simulink model "PropulsionTest"  (R2017b)
settings: Solver=FixedStepAuto  StartTime=0.0  StopTime=100*24*60*60  FixedStep=.2  RelTol=1e-3
model workspace: external: MATLAB File C:\Users\Justin\Documents\00 MEng Project\PAN_ADCS\initialization\simulink_workspace_init.m (data not in the file)
undefined symbols (not defined in the file): Imp_max, Imp_min, init, K_F, L_F, m_follower, match_tol, muE, ontime_max, ontime_min, Thrust_max, Thrust_min
libraries: hEemethod x8, vrlib x2, dspsigattribs x1
(part 1 of 2)
settings Model: Creator=Justin  LastModifiedBy=Justin

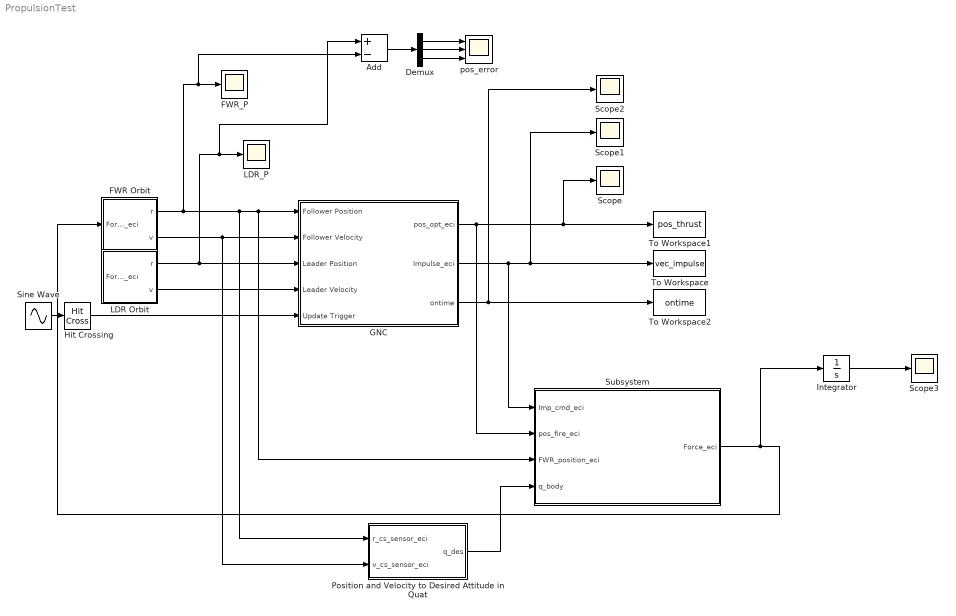
== system PropulsionTest ==
  Add : Sum  Inputs=+-
  Demux : Demux  Outputs=3
  FWR Orbit : Subsystem
  FWR_P : Scope
  GNC : Subsystem
  Hit Crossing : HitCross  HitCrossingOffset=0.5  HitCrossingDirection=rising
  Integrator : Integrator  InitialCondition=[0;0;0]
  LDR Orbit : Subsystem
  LDR_P : Scope
  Position and Velocity to Desired Attitude in Quat : Subsystem
  Scope{,1..3} (4 alike) : Scope
  Sine Wave : Sin  Frequency=2*pi/550  SampleTime=0
  Subsystem : Subsystem
  To Workspace : ToWorkspace  VariableName=vec_impulse  SaveFormat=Timeseries  SampleTime=-1
  To Workspace1 : ToWorkspace  VariableName=pos_thrust  SaveFormat=Timeseries  SampleTime=-1
  To Workspace2 : ToWorkspace  VariableName=ontime  SaveFormat=Timeseries  SampleTime=-1
  pos_error : Scope  NumInputPorts=3
  wires:
  Sine Wave/1 -> Hit Crossing/1
  GNC/3(ontime) -> Scope2/1, To Workspace2/1
  Hit Crossing/1 -> GNC/5(Update Trigger)
  GNC/1(pos_opt_eci) -> Scope/1, To Workspace1/1, Subsystem/2(pos_fire_eci)
  GNC/2(Impulse_eci) -> To Workspace/1, Scope1/1, Subsystem/1(Imp_cmd_eci)
  LDR Orbit/1(r) -> Add/1, LDR_P/1, GNC/3(Leader Position)
  LDR Orbit/2(v) -> GNC/4(Leader Velocity)
  FWR Orbit/2(v) -> Position and Velocity to Desired Attitude in Quat/2(v_cs_sensor_eci), GNC/2(Follower Velocity)
  FWR Orbit/1(r) -> Add/2, FWR_P/1, Position and Velocity to Desired Attitude in Quat/1(r_cs_sensor_eci), Subsystem/3(FWR_position_eci), GNC/1(Follower Position)
  Position and Velocity to Desired Attitude in Quat/1(q_des) -> Subsystem/4(q_body)
  Subsystem/1(Force_eci) -> FWR Orbit/1(Force_eci), Integrator/1
  Integrator/1 -> Scope3/1
  Add/1 -> Demux/1
  Demux/2 -> pos_error/2
  Demux/3 -> pos_error/3
  Demux/1 -> pos_error/1

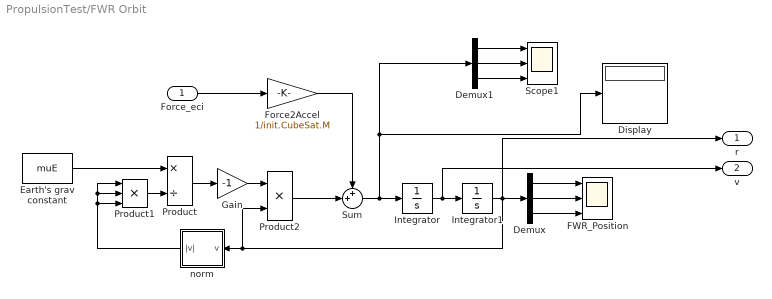
== system PropulsionTest/FWR Orbit ==
  Force_eci : Inport
  Demux : Demux  Outputs=3
  Demux1 : Demux  Outputs=3
  Display : Display
  Earth's grav constant : Constant  Value=muE
  FWR_Position : Scope  NumInputPorts=3
  Force2Accel : Gain  Gain=1/init.CubeSat.M
  Gain : Gain  Gain=-1  SaturateOnIntegerOverflow=on  OutDataTypeStr=Inherit: Same as input  ParamDataTypeStr=Inherit: Same as input
  Integrator : Integrator  InitialCondition=init.FWR.V
  Integrator1 : Integrator  InitialCondition=init.FWR.P
  Product : Product  Inputs=*/  SaturateOnIntegerOverflow=on  OutDataTypeStr=Inherit: Same as first input
  Product1 : Product  Inputs=***  SaturateOnIntegerOverflow=on  OutDataTypeStr=Inherit: Same as first input
  Product2 : Product  Inputs=**  SaturateOnIntegerOverflow=on  OutDataTypeStr=Inherit: Same as first input
  Scope1 : Scope  NumInputPorts=3
  Sum : Sum  Inputs=++|
  norm : Subsystem
  r : Outport
  v : Outport  Port=2
  wires:
  norm/1(|v|) -> Product1/3, Product1/2, Product1/1
  Demux/3 -> FWR_Position/3
  Demux/2 -> FWR_Position/2
  Demux/1 -> FWR_Position/1
  Gain/1 -> Product2/1
  Integrator/1 -> v/1, Integrator1/1
  Product/1 -> Gain/1
  Integrator1/1 -> r/1, Demux/1, norm/1(v), Product2/2
  Product1/1 -> Product/2
  Earth's grav constant/1 -> Product/1
  Force2Accel/1 -> Sum/1
  Product2/1 -> Sum/2
  Sum/1 -> Display/1, Demux1/1, Integrator/1
  Force_eci/1 -> Force2Accel/1
  Demux1/2 -> Scope1/2
  Demux1/3 -> Scope1/3
  Demux1/1 -> Scope1/1

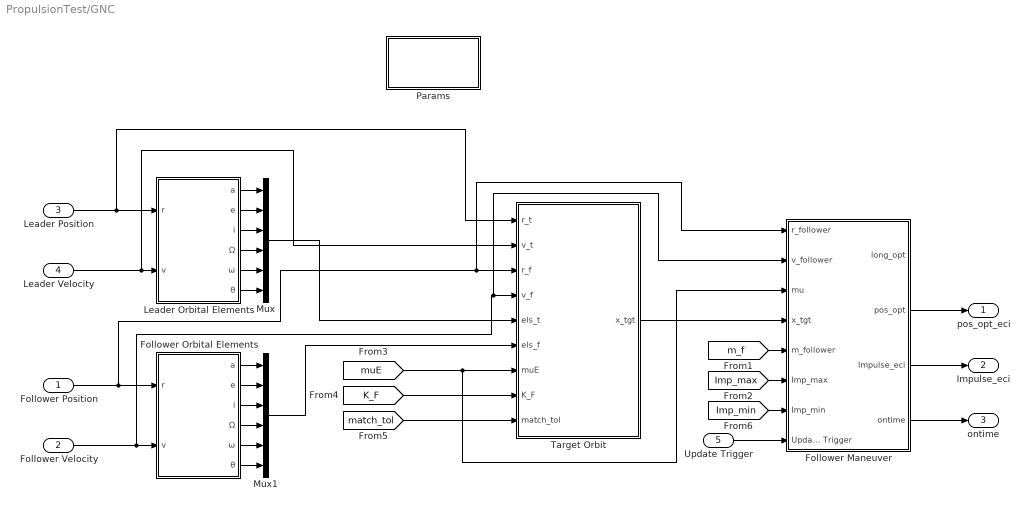
== system PropulsionTest/GNC ==
  Follower Position : Inport
  Follower Velocity : Inport  Port=2
  Leader Position : Inport  Port=3
  Leader Velocity : Inport  Port=4
  Update Trigger : Inport  Port=5
  Follower Maneuver : Subsystem
  Follower Orbital Elements : Subsystem
  Leader Orbital Elements : Subsystem
  Mux : Mux  Inputs=6
  Mux1 : Mux  Inputs=6
  Params : Subsystem
  Target Orbit : MATLAB Function  TreatAsAtomicUnit=on
  pos_opt_eci : Outport
  Impulse_eci : Outport  Port=2
  ontime : Outport  Port=3
  wires:
  Follower Position/1 -> Follower Orbital Elements/1(r), Follower Maneuver/1(r_follower), Target Orbit/3(r_f)
  Follower Maneuver/2(pos_opt) -> pos_opt_eci/1
  [Imp_min] -> Follower Maneuver/7(Imp_min)
  Follower Maneuver/3(Impulse_eci) -> Impulse_eci/1
  Leader Orbital Elements/4(Ω) -> Mux/4
  Mux/1 -> Target Orbit/5(els_t)
  Follower Orbital Elements/6(θ) -> Mux1/6
  Follower Orbital Elements/2(e) -> Mux1/2
  Follower Orbital Elements/3(i) -> Mux1/3
  Update Trigger/1 -> Follower Maneuver/8(Update Trigger)
  Leader Velocity/1 -> Leader Orbital Elements/2(v), Target Orbit/2(v_t)
  [Imp_max] -> Follower Maneuver/6(Imp_max)
  Target Orbit/1(x_tgt) -> Follower Maneuver/4(x_tgt)
  [muE] -> Follower Maneuver/3(mu), Target Orbit/7(muE)
  [match_tol] -> Target Orbit/9(match_tol)
  [m_f] -> Follower Maneuver/5(m_follower)
  Follower Velocity/1 -> Follower Orbital Elements/2(v), Follower Maneuver/2(v_follower), Target Orbit/4(v_f)
  Follower Orbital Elements/1(a) -> Mux1/1
  Follower Orbital Elements/4(Ω) -> Mux1/4
  Leader Orbital Elements/5(ω) -> Mux/5
  Follower Maneuver/4(ontime) -> ontime/1
  Mux1/1 -> Target Orbit/6(els_f)
  Leader Orbital Elements/3(i) -> Mux/3
  Follower Orbital Elements/5(ω) -> Mux1/5
  Leader Orbital Elements/6(θ) -> Mux/6
  Leader Position/1 -> Leader Orbital Elements/1(r), Target Orbit/1(r_t)
  Leader Orbital Elements/1(a) -> Mux/1
  Leader Orbital Elements/2(e) -> Mux/2
  [K_F] -> Target Orbit/8(K_F)

== system PropulsionTest/LDR Orbit ==
  Force_eci : Inport
  Demux : Demux  Outputs=3
  Earth's grav constant : Constant  Value=muE
  Force2Accel : Gain  Gain=1/init.CubeSat.M
  Gain : Gain  Gain=-1  SaturateOnIntegerOverflow=on  OutDataTypeStr=Inherit: Same as input  ParamDataTypeStr=Inherit: Same as input
  Integrator : Integrator  InitialCondition=init.LDR.V
  Integrator1 : Integrator  InitialCondition=init.LDR.P
  LDR_Position : Scope  NumInputPorts=3
  Product : Product  Inputs=*/  SaturateOnIntegerOverflow=on  OutDataTypeStr=Inherit: Same as first input
  Product1 : Product  Inputs=***  SaturateOnIntegerOverflow=on  OutDataTypeStr=Inherit: Same as first input
  Product2 : Product  Inputs=**  SaturateOnIntegerOverflow=on  OutDataTypeStr=Inherit: Same as first input
  Sum : Sum  Inputs=++|
  norm : Subsystem
  r : Outport
  v : Outport  Port=2
  wires:
  norm/1(|v|) -> Product1/3, Product1/2, Product1/1
  Demux/3 -> LDR_Position/3
  Demux/2 -> LDR_Position/2
  Demux/1 -> LDR_Position/1
  Gain/1 -> Product2/1
  Integrator/1 -> v/1, Integrator1/1
  Product/1 -> Gain/1
  Integrator1/1 -> r/1, Demux/1, norm/1(v), Product2/2
  Product1/1 -> Product/2
  Earth's grav constant/1 -> Product/1
  Force2Accel/1 -> Sum/1
  Product2/1 -> Sum/2
  Sum/1 -> Integrator/1
  Force_eci/1 -> Force2Accel/1

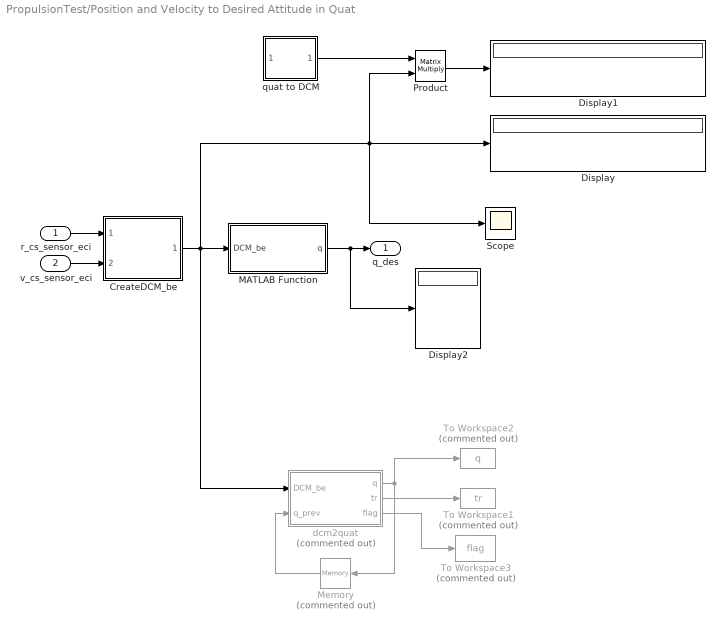
== system PropulsionTest/Position and Velocity to Desired Attitude in Quat ==
  r_cs_sensor_eci : Inport
  v_cs_sensor_eci : Inport  Port=2
  CreateDCM_be : Subsystem
  Display : Display
  Display1 : Display
  Display2 : Display
  MATLAB Function : MATLAB Function  TreatAsAtomicUnit=on
  Memory : Memory  Commented=on
  Product : Product  Multiplication=Matrix(*)
  Scope : Scope
  To Workspace1 : ToWorkspace  Commented=on  VariableName=tr  SampleTime=-1
  To Workspace2 : ToWorkspace  Commented=on  VariableName=q  SampleTime=-1
  To Workspace3 : ToWorkspace  Commented=on  VariableName=flag  SampleTime=-1
  dcm2quat : MATLAB Function  Commented=on  TreatAsAtomicUnit=on
  quat to DCM : Subsystem  mask(Direction Cosine Matrix){}
      mask help: Determines the 3x3 Direction Cosine Matrix (DCM) from a 4x1 quaternion orientation vector. The outputted DCM transforms vectors from inertial axes to body axes. This version corrects the fucked-up MATLAB one.
      mask Help:
      | <p>This block determines the 3x3 Direction Cosine Matrix (DCM) from a 4x1 quaternion orientation vector. The outputted DCM transforms vectors from inertial axes to body axes.  This version corrects the fucked-up MATLAB one</p>
      | 
      | <p>The block input and output contain more than one signal as described below.</p>
      | 
      | <p><H4>Block Vector Input - Quaternion</H4>
      | <ul>
      | <li>q0</li>
      | <li>q1</li>
      | <li>q2</li>
      | <li>q3</li>
      | </ul>
      | </p>
      | 
      | <p><H4>Block Matrix Output - Direction Cosine Matrix  </H4>
      |     <ul>
      |    </ul>
      |    </p>
      mask Display: disp('q to Q')
  q_des : Outport
  wires:
  r_cs_sensor_eci/1 -> CreateDCM_be/1(Position)
  v_cs_sensor_eci/1 -> CreateDCM_be/2(Velocity)
  dcm2quat/1(q) -> Memory/1, To Workspace2/1
  CreateDCM_be/1(DCM_be) -> dcm2quat/1(DCM_be), MATLAB Function/1(DCM_be), Scope/1, Product/2, Display/1
  dcm2quat/2(tr) -> To Workspace1/1
  dcm2quat/3(flag) -> To Workspace3/1
  Memory/1 -> dcm2quat/2(q_prev)
  Product/1 -> Display1/1
  quat to DCM/1(DCM) -> Product/1
  MATLAB Function/1(q) -> Display2/1, q_des/1

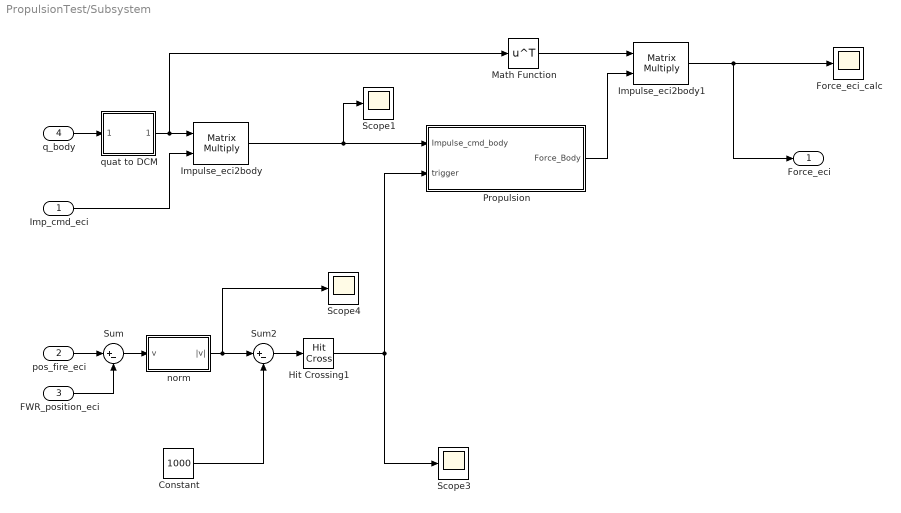
== system PropulsionTest/Subsystem ==
  Imp_cmd_eci : Inport
  pos_fire_eci : Inport  Port=2
  FWR_position_eci : Inport  Port=3
  q_body : Inport  Port=4
  Constant : Constant  Value=1000
  Force_eci_calc : Scope
  Hit Crossing1 : HitCross  HitCrossingDirection=falling
  Impulse_eci2body : Product  Multiplication=Matrix(*)
  Impulse_eci2body1 : Product  Multiplication=Matrix(*)
  Math Function : Math  Operator=transpose  SaturateOnIntegerOverflow=on
  Propulsion : Subsystem
  Scope1 : Scope
  Scope3 : Scope
  Scope4 : Scope
  Sum : Sum  Inputs=|+-
  Sum2 : Sum  Inputs=|+-
  norm : Subsystem
  quat to DCM : Subsystem  mask(Direction Cosine Matrix){}
      mask help: Determines the 3x3 Direction Cosine Matrix (DCM) from a 4x1 quaternion orientation vector. The outputted DCM transforms vectors from inertial axes to body axes. This version corrects the fucked-up MATLAB one.
      mask Help:
      | <p>This block determines the 3x3 Direction Cosine Matrix (DCM) from a 4x1 quaternion orientation vector. The outputted DCM transforms vectors from inertial axes to body axes.  This version corrects the fucked-up MATLAB one</p>
      | 
      | <p>The block input and output contain more than one signal as described below.</p>
      | 
      | <p><H4>Block Vector Input - Quaternion</H4>
      | <ul>
      | <li>q0</li>
      | <li>q1</li>
      | <li>q2</li>
      | <li>q3</li>
      | </ul>
      | </p>
      | 
      | <p><H4>Block Matrix Output - Direction Cosine Matrix  </H4>
      |     <ul>
      |    </ul>
      |    </p>
      mask Display: disp('q to Q')
  Force_eci : Outport
  wires:
  pos_fire_eci/1 -> Sum/1
  FWR_position_eci/1 -> Sum/2
  Sum2/1 -> Hit Crossing1/1
  norm/1(|v|) -> Sum2/1, Scope4/1
  Constant/1 -> Sum2/2
  Sum/1 -> norm/1(v)
  Imp_cmd_eci/1 -> Impulse_eci2body/2
  q_body/1 -> quat to DCM/1(e0 e1 e2 e3)
  Impulse_eci2body/1 -> Scope1/1, Propulsion/1(Impulse_cmd_body)
  Hit Crossing1/1 -> Propulsion/2(trigger), Scope3/1
  Propulsion/1(Force_Body) -> Impulse_eci2body1/2
  quat to DCM/1(DCM) -> Math Function/1, Impulse_eci2body/1
  Math Function/1 -> Impulse_eci2body1/1
  Impulse_eci2body1/1 -> Force_eci/1, Force_eci_calc/1

== system PropulsionTest/FWR Orbit/norm ==
  v : Inport
  Dot Product : DotProduct  InputSameDT=on  OutDataTypeStr=Inherit: Inherit via internal rule
  Math Function : Math  Operator=sqrt  SaturateOnIntegerOverflow=on
  Saturation : Saturate  UpperLimit=1e20  LowerLimit=1e-10
  |v| : Outport
  wires:
  Saturation/1 -> |v|/1
  Math Function/1 -> Saturation/1
  Dot Product/1 -> Math Function/1
  v/1 -> Dot Product/2, Dot Product/1

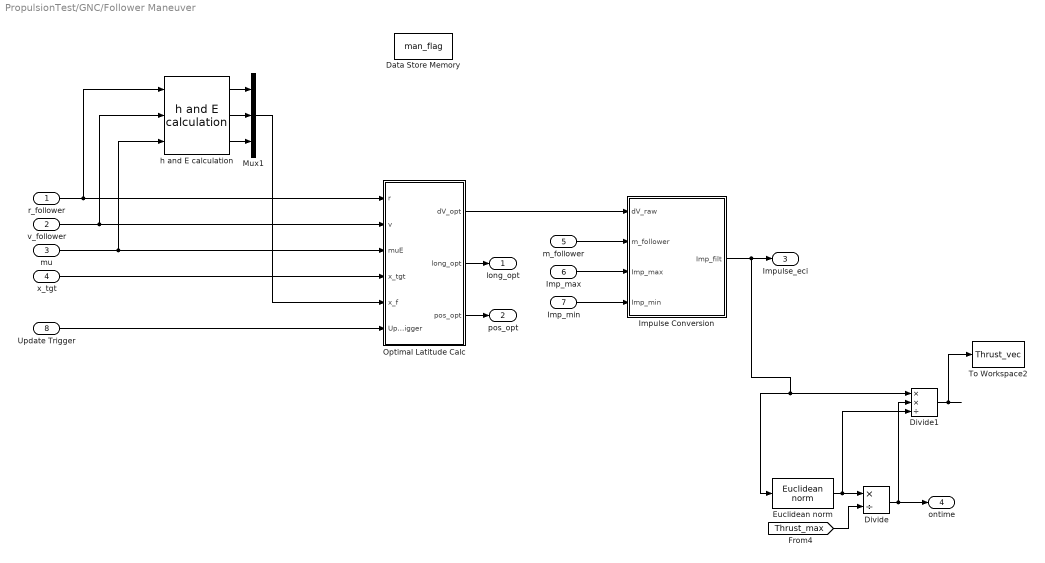
== system PropulsionTest/GNC/Follower Maneuver ==
  r_follower : Inport
  v_follower : Inport  Port=2
  mu : Inport  Port=3
  x_tgt : Inport  Port=4
  m_follower : Inport  Port=5
  Imp_max : Inport  Port=6
  Imp_min : Inport  Port=7
  Update Trigger : Inport  Port=8
  Data Store Memory : DataStoreMemory  DataStoreName=man_flag  WriteAfterWriteMsg=warning  WriteAfterReadMsg=warning  ShowAdditionalParam=off
  Divide : Product  Inputs=*/
  Divide1 : Product  Inputs=**/
  Euclidean norm : hEemethod/Math Operations/Euclidean norm
      settings: SourceProductName=HEe Method Library
  Impulse Conversion : MATLAB Function  TreatAsAtomicUnit=on
  Mux1 : Mux  Inputs=3
  Optimal Latitude Calc : Subsystem
  To Workspace2 : ToWorkspace  VariableName=Thrust_vec  SaveFormat=Timeseries  SampleTime=-1
  h and E calculation : hEemethod/Math Operations/h and E calculation
      settings: SourceProductName=HEe Method Library
  long_opt : Outport
  pos_opt : Outport  Port=2
  Impulse_eci : Outport  Port=3
  ontime : Outport  Port=4
  wires:
  r_follower/1 -> h and E calculation/1, Optimal Latitude Calc/1("r ")
  h and E calculation/1 -> Mux1/1
  h and E calculation/2 -> Mux1/2
  Mux1/1 -> Optimal Latitude Calc/5(x_f)
  x_tgt/1 -> Optimal Latitude Calc/4(x_tgt)
  mu/1 -> h and E calculation/3, Optimal Latitude Calc/3(muE)
  v_follower/1 -> h and E calculation/2, Optimal Latitude Calc/2("v ")
  h and E calculation/3 -> Mux1/3
  Optimal Latitude Calc/2(long_opt) -> long_opt/1
  Optimal Latitude Calc/1(dV_opt) -> Impulse Conversion/1(dV_raw)
  Imp_min/1 -> Impulse Conversion/4(Imp_min)
  Imp_max/1 -> Impulse Conversion/3(Imp_max)
  m_follower/1 -> Impulse Conversion/2(m_follower)
  Update Trigger/1 -> Optimal Latitude Calc/6(Update Trigger)
  Optimal Latitude Calc/3(pos_opt) -> pos_opt/1
  Euclidean norm/1 -> Divide1/3, Divide/1
  Divide1/1 -> To Workspace2/1
  [Thrust_max] -> Divide/2
  Divide/1 -> Divide1/2, ontime/1
  Impulse Conversion/1(Imp_filt) -> Euclidean norm/1, Divide1/1, Impulse_eci/1

== system PropulsionTest/GNC/Follower Orbital Elements ==
  r : Inport
  v : Inport  Port=2
  Follower True Anomaly : hEemethod/Math Operations/True Anomaly
      settings: SourceProductName=HEe Method Library
  Mux : Mux  Inputs=3
  Orbital Elements : hEemethod/Math Operations/Orbital Elements
      settings: SourceProductName=HEe Method Library
  h and E calculation : hEemethod/Math Operations/h and E calculation
      settings: SourceProductName=HEe Method Library
  a : Outport
  e : Outport  Port=2
  i : Outport  Port=3
  Ω : Outport  Port=4
  ω : Outport  Port=5
  θ : Outport  Port=6
  wires:
  h and E calculation/1 -> Mux/1
  Orbital Elements/5 -> ω/1
  Orbital Elements/2 -> e/1
  Orbital Elements/3 -> i/1
  Orbital Elements/1 -> a/1
  r/1 -> Follower True Anomaly/1, h and E calculation/1
  Orbital Elements/4 -> Ω/1
  v/1 -> Follower True Anomaly/2, h and E calculation/2
  Mux/1 -> Orbital Elements/1
  h and E calculation/2 -> Mux/2
  h and E calculation/3 -> Mux/3
  [muE] -> Follower True Anomaly/3, Orbital Elements/2, h and E calculation/3
  Follower True Anomaly/1 -> θ/1

== system PropulsionTest/GNC/Leader Orbital Elements ==
  r : Inport
  v : Inport  Port=2
  Follower True Anomaly : hEemethod/Math Operations/True Anomaly
      settings: SourceProductName=HEe Method Library
  Mux : Mux  Inputs=3
  Orbital Elements : hEemethod/Math Operations/Orbital Elements
      settings: SourceProductName=HEe Method Library
  h and E calculation : hEemethod/Math Operations/h and E calculation
      settings: SourceProductName=HEe Method Library
  a : Outport
  e : Outport  Port=2
  i : Outport  Port=3
  Ω : Outport  Port=4
  ω : Outport  Port=5
  θ : Outport  Port=6
  wires:
  h and E calculation/1 -> Mux/1
  Orbital Elements/5 -> ω/1
  Orbital Elements/2 -> e/1
  Orbital Elements/3 -> i/1
  Orbital Elements/1 -> a/1
  r/1 -> Follower True Anomaly/1, h and E calculation/1
  Orbital Elements/4 -> Ω/1
  v/1 -> Follower True Anomaly/2, h and E calculation/2
  Mux/1 -> Orbital Elements/1
  h and E calculation/2 -> Mux/2
  h and E calculation/3 -> Mux/3
  [muE] -> Follower True Anomaly/3, Orbital Elements/2, h and E calculation/3
  Follower True Anomaly/1 -> θ/1

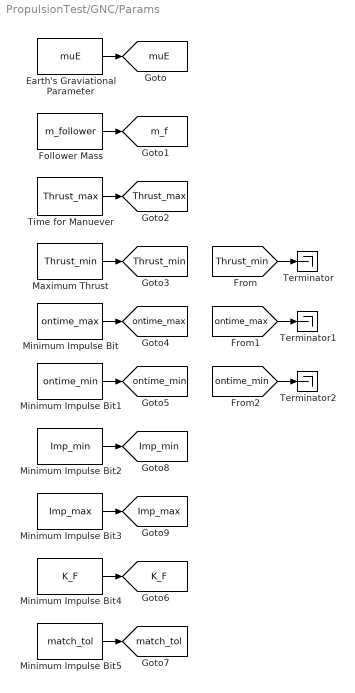
== system PropulsionTest/GNC/Params ==
  Earth's Graviational Parameter : Constant  Value=muE
  Follower Mass : Constant  Value=m_follower
  Maximum Thrust : Constant  Value=Thrust_min
  Minimum Impulse Bit : Constant  Value=ontime_max
  Minimum Impulse Bit1 : Constant  Value=ontime_min
  Minimum Impulse Bit2 : Constant  Value=Imp_min
  Minimum Impulse Bit3 : Constant  Value=Imp_max
  Minimum Impulse Bit4 : Constant  Value=K_F
  Minimum Impulse Bit5 : Constant  Value=match_tol
  Terminator : Terminator
  Terminator1 : Terminator
  Terminator2 : Terminator
  Time for Manuever : Constant  Value=Thrust_max
  tag scope: Imp_max=global, Imp_min=global, K_F=global, Thrust_max=global, Thrust_min=global, m_f=global, match_tol=global, muE=global, ontime_max=global, ontime_min=global
  wires:
  Time for Manuever/1 -> [Thrust_max]
  Follower Mass/1 -> [m_f]
  Earth's Graviational Parameter/1 -> [muE]
  Maximum Thrust/1 -> [Thrust_min]
  Minimum Impulse Bit/1 -> [ontime_max]
  Minimum Impulse Bit1/1 -> [ontime_min]
  Minimum Impulse Bit2/1 -> [Imp_min]
  Minimum Impulse Bit3/1 -> [Imp_max]
  [Thrust_min] -> Terminator/1
  [ontime_max] -> Terminator1/1
  [ontime_min] -> Terminator2/1
  Minimum Impulse Bit4/1 -> [K_F]
  Minimum Impulse Bit5/1 -> [match_tol]

== system PropulsionTest/LDR Orbit/norm ==
  v : Inport
  Dot Product : DotProduct  InputSameDT=on  OutDataTypeStr=Inherit: Inherit via internal rule
  Math Function : Math  Operator=sqrt  SaturateOnIntegerOverflow=on
  Saturation : Saturate  UpperLimit=1e20  LowerLimit=1e-10
  |v| : Outport
  wires:
  Saturation/1 -> |v|/1
  Math Function/1 -> Saturation/1
  Dot Product/1 -> Math Function/1
  v/1 -> Dot Product/2, Dot Product/1

== system PropulsionTest/Position and Velocity to Desired Attitude in Quat/CreateDCM_be ==
  Position : Inport
  Velocity : Inport  Port=2
  Cross Product : vrlib/Utilities/Cross Product
      settings: SourceProductBaseCode=VR
  Cross Product1 : vrlib/Utilities/Cross Product
      settings: SourceProductBaseCode=VR
  Matrix Concatenate : Concatenate  NumInputs=3  Mode=Multidimensional array  ConcatenateDimension=2
  normalize : Subsystem
  normalize2 : Subsystem
  DCM_be : Outport
  wires:
  normalize/1(r_hat) -> Cross Product1/1, Matrix Concatenate/1
  Cross Product/1 -> normalize2/1(v)
  Velocity/1 -> Cross Product/1
  Matrix Concatenate/1 -> DCM_be/1
  Position/1 -> Cross Product/2, normalize/1(r)
  Cross Product1/1 -> Matrix Concatenate/3
  normalize2/1(v_hat) -> Cross Product1/2, Matrix Concatenate/2

== system PropulsionTest/Position and Velocity to Desired Attitude in Quat/quat to DCM ==
  e0 e1 e2 e3 : Inport
  Demux : Demux
  Gain1 : Gain  Gain=2  SaturateOnIntegerOverflow=on  OutDataTypeStr=Inherit: Same as input  ParamDataTypeStr=Inherit: Same as input
  Gain2 : Gain  Gain=2  SaturateOnIntegerOverflow=on  OutDataTypeStr=Inherit: Same as input  ParamDataTypeStr=Inherit: Same as input
  Matrix Gain : Gain  Gain=eye(3,3)  SaturateOnIntegerOverflow=on  OutDataTypeStr=Inherit: Same as input  ParamDataTypeStr=Inherit: Same as input
  Mux : Mux  Inputs=3
  Product : Product  SaturateOnIntegerOverflow=on  InputSameDT=on  OutDataTypeStr=Inherit: Same as first input
  Product1 : Product  SaturateOnIntegerOverflow=on  InputSameDT=on  OutDataTypeStr=Inherit: Same as first input
  Subsystem : Subsystem
      mask Display: disp('3x3 cross matrix')
  Sum1 : Sum  Inputs=|+-  SaturateOnIntegerOverflow=on  InputSameDT=on  OutDataTypeStr=Inherit: Same as first input
  Sum8 : Sum  Inputs=|+-+  SaturateOnIntegerOverflow=on  InputSameDT=on  OutDataTypeStr=Inherit: Same as first input
  T1 : Math  Operator=transpose  SaturateOnIntegerOverflow=on
  T2 : Math  Operator=transpose  SaturateOnIntegerOverflow=on
  qTq : Product  Multiplication=Matrix(*)  SaturateOnIntegerOverflow=on  InputSameDT=on  OutDataTypeStr=Inherit: Same as first input
  qqT : Product  Multiplication=Matrix(*)  SaturateOnIntegerOverflow=on  InputSameDT=on  OutDataTypeStr=Inherit: Same as first input
  DCM : Outport  InitialOutput=0
  wires:
  Subsystem/1(Out1) -> Product/1
  Matrix Gain/1 -> Sum8/3
  Sum1/1 -> Matrix Gain/1
  qTq/1 -> Sum1/2
  T2/1 -> qTq/1
  Product1/1 -> Sum1/1
  Gain1/1 -> Sum8/2
  Gain2/1 -> Sum8/1
  qqT/1 -> Gain2/1
  T1/1 -> qqT/2
  Product/1 -> Gain1/1
  Mux/1 -> qTq/2, T2/1, qqT/1, T1/1, Subsystem/1(In1)
  Demux/4 -> Product1/2, Product1/1, Product/2
  Demux/3 -> Mux/3
  Demux/2 -> Mux/2
  Demux/1 -> Mux/1
  e0 e1 e2 e3/1 -> Demux/1
  Sum8/1 -> DCM/1

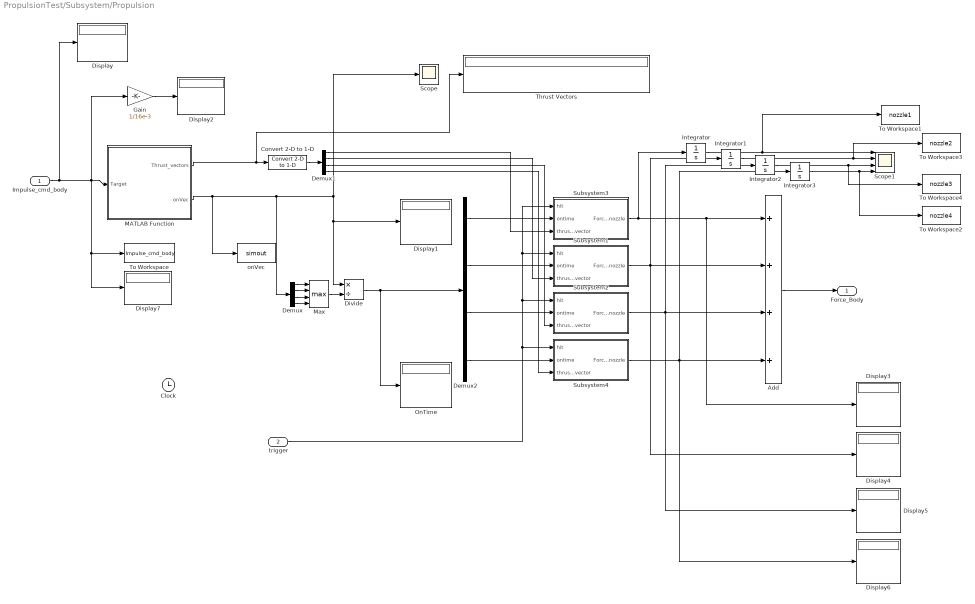
== system PropulsionTest/Subsystem/Propulsion ==
  Impulse_cmd_body : Inport
  trigger : Inport  Port=2
  Add : Sum  Inputs=++++
  Clock : Clock
  Convert 2-D to 1-D : dspsigattribs/Convert 2-D to 1-D
      settings: SourceProductName=DSP System Toolbox  SourceProductBaseCode=DS
  Demux : Demux
  Demux1 : Demux
  Demux2 : Demux
  Display{,1..7} (8 alike) : Display
  Divide : Product  Inputs=*/
  Gain : Gain  Gain=1/16e-3
  Integrator{,1..3} (4 alike) : Integrator  InitialCondition=[0;0;0]
  MATLAB Function : MATLAB Function  TreatAsAtomicUnit=on
  Max : MinMax  Function=max  Inputs=4
  OnTime : Display
  Scope : Scope
  Scope1 : Scope  NumInputPorts=4
  Subsystem1 : Subsystem
  Subsystem2 : Subsystem
  Subsystem3 : Subsystem
  Subsystem4 : Subsystem
  Thrust Vectors : Display
  To Workspace : ToWorkspace  VariableName=Impulse_cmd_body  SaveFormat=Timeseries  SampleTime=-1
  To Workspace1 : ToWorkspace  VariableName=nozzle1  SaveFormat=Timeseries  SampleTime=-1
  To Workspace2 : ToWorkspace  VariableName=nozzle4  SaveFormat=Timeseries  SampleTime=-1
  To Workspace3 : ToWorkspace  VariableName=nozzle2  SaveFormat=Timeseries  SampleTime=-1
  To Workspace4 : ToWorkspace  VariableName=nozzle3  SaveFormat=Timeseries  SampleTime=-1
  onVec : ToWorkspace  VariableName=simout  SaveFormat=Timeseries  SampleTime=-1
  Force_Body : Outport
  wires:
  Impulse_cmd_body/1 -> Display/1, Display7/1, To Workspace/1, Gain/1, MATLAB Function/1(Target)
  MATLAB Function/2(onVec) -> onVec/1, Demux/1, Divide/1, Display1/1, Scope/1
  trigger/1 -> Subsystem4/1(hit), Subsystem2/1(hit), Subsystem1/1(hit), Subsystem3/1(hit)
  Gain/1 -> Display2/1
  Max/1 -> Divide/2
  Divide/1 -> OnTime/1, Demux2/1
  Demux/1 -> Max/1
  Demux/2 -> Max/2
  Demux/3 -> Max/3
  Demux/4 -> Max/4
  Convert 2-D to 1-D/1 -> Demux1/1
  MATLAB Function/1(Thrust_vectors) -> Thrust Vectors/1, Convert 2-D to 1-D/1
  Demux2/1 -> Subsystem3/2(ontime)
  Demux2/2 -> Subsystem1/2(ontime)
  Demux2/3 -> Subsystem2/2(ontime)
  Demux2/4 -> Subsystem4/2(ontime)
  Demux1/1 -> Subsystem3/3(thrust_vector)
  Demux1/2 -> Subsystem1/3(thrust_vector)
  Demux1/3 -> Subsystem2/3(thrust_vector)
  Demux1/4 -> Subsystem4/3(thrust_vector)
  Subsystem3/1(Force_nozzle) -> Integrator/1, Display3/1, Add/1
  Subsystem4/1(Force_nozzle) -> Display6/1, Add/4, Integrator3/1
  Subsystem2/1(Force_nozzle) -> Display5/1, Add/3, Integrator2/1
  Subsystem1/1(Force_nozzle) -> Display4/1, Add/2, Integrator1/1
  Add/1 -> Force_Body/1
  Integrator/1 -> To Workspace1/1, Scope1/1
  Integrator1/1 -> To Workspace3/1, Scope1/2
  Integrator2/1 -> To Workspace4/1, Scope1/3
  Integrator3/1 -> To Workspace2/1, Scope1/4

== system PropulsionTest/Subsystem/norm ==
  v : Inport
  Dot Product : DotProduct  InputSameDT=on  OutDataTypeStr=Inherit: Inherit via internal rule
  Math Function : Math  Operator=sqrt  SaturateOnIntegerOverflow=on
  |v| : Outport
  wires:
  Math Function/1 -> |v|/1
  Dot Product/1 -> Math Function/1
  v/1 -> Dot Product/2, Dot Product/1

== system PropulsionTest/Subsystem/quat to DCM ==
  e0 e1 e2 e3 : Inport
  Demux : Demux
  Gain1 : Gain  Gain=2  SaturateOnIntegerOverflow=on  OutDataTypeStr=Inherit: Same as input  ParamDataTypeStr=Inherit: Same as input
  Gain2 : Gain  Gain=2  SaturateOnIntegerOverflow=on  OutDataTypeStr=Inherit: Same as input  ParamDataTypeStr=Inherit: Same as input
  Matrix Gain : Gain  Gain=eye(3,3)  SaturateOnIntegerOverflow=on  OutDataTypeStr=Inherit: Same as input  ParamDataTypeStr=Inherit: Same as input
  Mux : Mux  Inputs=3
  Product : Product  SaturateOnIntegerOverflow=on  InputSameDT=on  OutDataTypeStr=Inherit: Same as first input
  Product1 : Product  SaturateOnIntegerOverflow=on  InputSameDT=on  OutDataTypeStr=Inherit: Same as first input
  Subsystem : Subsystem
      mask Display: disp('3x3 cross matrix')
  Sum1 : Sum  Inputs=|+-  SaturateOnIntegerOverflow=on  InputSameDT=on  OutDataTypeStr=Inherit: Same as first input
  Sum8 : Sum  Inputs=|+-+  SaturateOnIntegerOverflow=on  InputSameDT=on  OutDataTypeStr=Inherit: Same as first input
  T1 : Math  Operator=transpose  SaturateOnIntegerOverflow=on
  T2 : Math  Operator=transpose  SaturateOnIntegerOverflow=on
  qTq : Product  Multiplication=Matrix(*)  SaturateOnIntegerOverflow=on  InputSameDT=on  OutDataTypeStr=Inherit: Same as first input
  qqT : Product  Multiplication=Matrix(*)  SaturateOnIntegerOverflow=on  InputSameDT=on  OutDataTypeStr=Inherit: Same as first input
  DCM : Outport  InitialOutput=0
  wires:
  Sum8/1 -> DCM/1
  e0 e1 e2 e3/1 -> Demux/1
  Demux/1 -> Mux/1
  Demux/2 -> Mux/2
  Demux/3 -> Mux/3
  Demux/4 -> Product/2, Product1/1, Product1/2
  Mux/1 -> T1/1, qqT/1, Subsystem/1(In1), T2/1, qTq/2
  Product/1 -> Gain1/1
  T1/1 -> qqT/2
  qqT/1 -> Gain2/1
  Gain2/1 -> Sum8/1
  Gain1/1 -> Sum8/2
  Product1/1 -> Sum1/1
  T2/1 -> qTq/1
  qTq/1 -> Sum1/2
  Sum1/1 -> Matrix Gain/1
  Matrix Gain/1 -> Sum8/3
  Subsystem/1(Out1) -> Product/1

== system PropulsionTest/GNC/Follower Maneuver/Optimal Latitude Calc ==
  "r " : Inport
  "v " : Inport  Port=2
  muE : Inport  Port=3
  x_tgt : Inport  Port=4
  x_f : Inport  Port=5
  Update Trigger : Inport  Port=6
  Constant : Constant  Value=K_F
  Constant1 : Constant  Value=L_F
  Enabled Subsystem : Subsystem  TreatAsAtomicUnit=on
  dV_opt : Outport
  long_opt : Outport  Port=2
  pos_opt : Outport  Port=3
  wires:
  Enabled Subsystem/2(long_opt) -> long_opt/1
  "r "/1 -> Enabled Subsystem/1(r)
  "v "/1 -> Enabled Subsystem/2(v)
  muE/1 -> Enabled Subsystem/7("muE ")
  x_tgt/1 -> Enabled Subsystem/3(x_tgt)
  x_f/1 -> Enabled Subsystem/4(x_f)
  Constant/1 -> Enabled Subsystem/5(K)
  Constant1/1 -> Enabled Subsystem/6(L)
  Enabled Subsystem/1(dV_opt) -> dV_opt/1
  Enabled Subsystem/3(pos_opt) -> pos_opt/1
  Update Trigger/1 -> Enabled Subsystem/Enable

== system PropulsionTest/Position and Velocity to Desired Attitude in Quat/CreateDCM_be/normalize ==
  r : Inport
  Dot Product : DotProduct  InputSameDT=on  OutDataTypeStr=Inherit: Inherit via internal rule
  Math Function : Math  Operator=sqrt  SaturateOnIntegerOverflow=on
  Product : Product  Inputs=*/  SaturateOnIntegerOverflow=on  InputSameDT=on  OutDataTypeStr=Inherit: Same as first input
  r_hat : Outport
  wires:
  r/1 -> Dot Product/1, Dot Product/2, Product/1
  Dot Product/1 -> Math Function/1
  Math Function/1 -> Product/2
  Product/1 -> r_hat/1

== system PropulsionTest/Position and Velocity to Desired Attitude in Quat/CreateDCM_be/normalize2 ==
  v : Inport
  Dot Product : DotProduct  InputSameDT=on  OutDataTypeStr=Inherit: Inherit via internal rule
  Math Function : Math  Operator=sqrt  SaturateOnIntegerOverflow=on
  Product : Product  Inputs=*/  SaturateOnIntegerOverflow=on  InputSameDT=on  OutDataTypeStr=Inherit: Same as first input
  v_hat : Outport
  wires:
  v/1 -> Dot Product/1, Dot Product/2, Product/1
  Dot Product/1 -> Math Function/1
  Math Function/1 -> Product/2
  Product/1 -> v_hat/1

== system PropulsionTest/Position and Velocity to Desired Attitude in Quat/quat to DCM/Subsystem ==
  In1 : Inport
  3x3 : Reshape  OutputDimensionality=Customize  OutputDimensions=[3,3]
  Demux : Demux  Outputs=3
  Gain : Gain  Gain=-1  SaturateOnIntegerOverflow=on  OutDataTypeStr=Inherit: Same as input  ParamDataTypeStr=Inherit: Same as input
  Gain1 : Gain  Gain=-1  SaturateOnIntegerOverflow=on  OutDataTypeStr=Inherit: Same as input  ParamDataTypeStr=Inherit: Same as input
  Gain2 : Gain  Gain=-1  SaturateOnIntegerOverflow=on  OutDataTypeStr=Inherit: Same as input  ParamDataTypeStr=Inherit: Same as input
  Mux : Mux  Inputs=9
  "diag 0 " : Constant  Value=0
  Out1 : Outport
  wires:
  Gain2/1 -> Mux/8
  Demux/1 -> Gain2/1, Mux/6
  Gain1/1 -> Mux/4
  Demux/2 -> Mux/7, Gain/1
  Gain/1 -> Mux/3
  Demux/3 -> Gain1/1, Mux/2
  Mux/1 -> 3x3/1
  "diag 0 "/1 -> Mux/9, Mux/5, Mux/1
  3x3/1 -> Out1/1
  In1/1 -> Demux/1

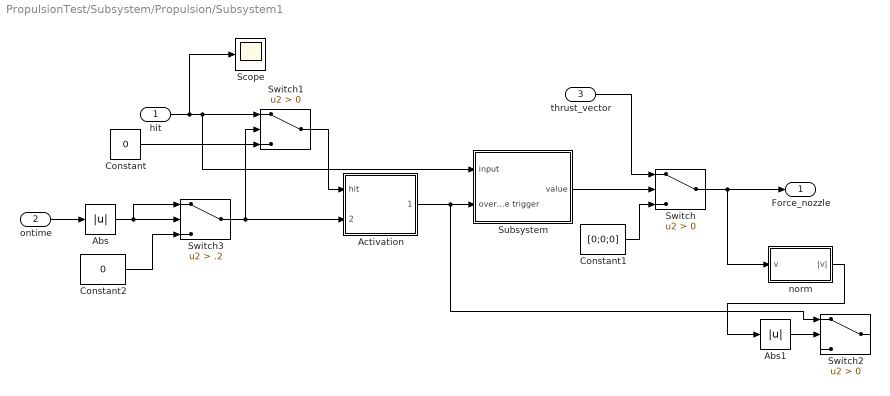
== system PropulsionTest/Subsystem/Propulsion/Subsystem1 ==
  hit : Inport
  ontime : Inport  Port=2
  thrust_vector : Inport  Port=3
  Abs : Abs
  Abs1 : Abs
  Activation : Subsystem
  Constant : Constant  Value=0
  Constant1 : Constant  Value=[0;0;0]
  Constant2 : Constant  Value=0
  Scope : Scope
  Subsystem : Subsystem
  Switch : Switch  Criteria=u2 > Threshold
  Switch1 : Switch  Criteria=u2 > Threshold
  Switch2 : Switch  Criteria=u2 > Threshold
  Switch3 : Switch  Criteria=u2 > Threshold  Threshold=.2
  norm : Subsystem
  Force_nozzle : Outport
  wires:
  Switch3/1 -> Switch1/2, Activation/2(T_maneuver)
  Constant2/1 -> Switch3/3
  ontime/1 -> Abs/1
  hit/1 -> Scope/1, Subsystem/1(input), Switch1/1
  Switch/1 -> norm/1(v), Force_nozzle/1
  Activation/1(man_end) -> Switch2/1, Subsystem/2(overwrite trigger)
  thrust_vector/1 -> Switch/1
  Subsystem/1(value) -> Switch/2
  Constant1/1 -> Switch/3
  Abs/1 -> Switch3/2, Switch3/1
  Switch1/1 -> Activation/1(hit)
  Constant/1 -> Switch1/3
  Abs1/1 -> Switch2/2
  norm/1(|v|) -> Abs1/1

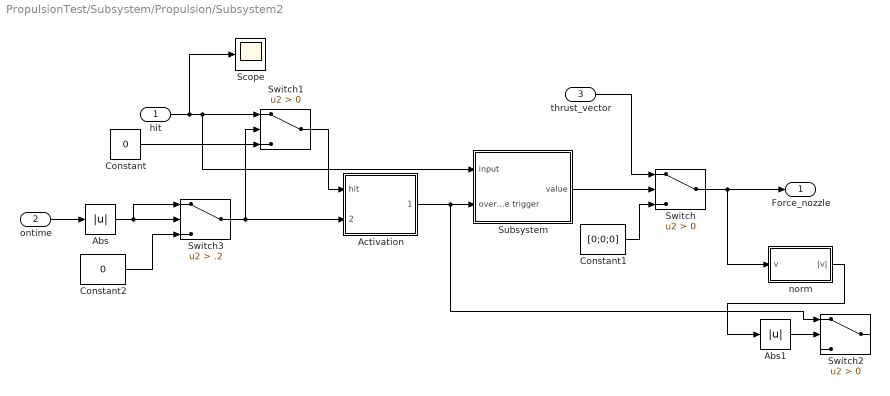
== system PropulsionTest/Subsystem/Propulsion/Subsystem2 ==
  hit : Inport
  ontime : Inport  Port=2
  thrust_vector : Inport  Port=3
  Abs : Abs
  Abs1 : Abs
  Activation : Subsystem
  Constant : Constant  Value=0
  Constant1 : Constant  Value=[0;0;0]
  Constant2 : Constant  Value=0
  Scope : Scope
  Subsystem : Subsystem
  Switch : Switch  Criteria=u2 > Threshold
  Switch1 : Switch  Criteria=u2 > Threshold
  Switch2 : Switch  Criteria=u2 > Threshold
  Switch3 : Switch  Criteria=u2 > Threshold  Threshold=.2
  norm : Subsystem
  Force_nozzle : Outport
  wires:
  norm/1(|v|) -> Abs1/1
  Abs1/1 -> Switch2/2
  Constant/1 -> Switch1/3
  Switch1/1 -> Activation/1(hit)
  Abs/1 -> Switch3/1, Switch3/2
  Constant1/1 -> Switch/3
  Subsystem/1(value) -> Switch/2
  thrust_vector/1 -> Switch/1
  Activation/1(man_end) -> Subsystem/2(overwrite trigger), Switch2/1
  Switch/1 -> Force_nozzle/1, norm/1(v)
  hit/1 -> Switch1/1, Subsystem/1(input), Scope/1
  ontime/1 -> Abs/1
  Constant2/1 -> Switch3/3
  Switch3/1 -> Activation/2(T_maneuver), Switch1/2

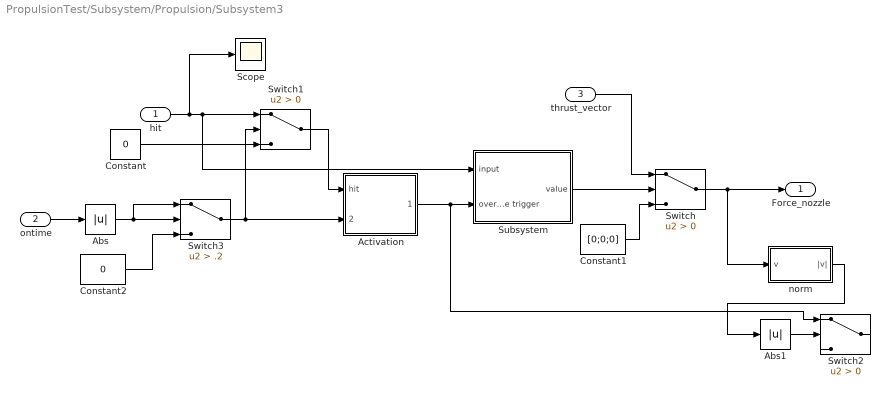
== system PropulsionTest/Subsystem/Propulsion/Subsystem3 ==
  hit : Inport
  ontime : Inport  Port=2
  thrust_vector : Inport  Port=3
  Abs : Abs
  Abs1 : Abs
  Activation : Subsystem
  Constant : Constant  Value=0
  Constant1 : Constant  Value=[0;0;0]
  Constant2 : Constant  Value=0
  Scope : Scope
  Subsystem : Subsystem
  Switch : Switch  Criteria=u2 > Threshold
  Switch1 : Switch  Criteria=u2 > Threshold
  Switch2 : Switch  Criteria=u2 > Threshold
  Switch3 : Switch  Criteria=u2 > Threshold  Threshold=.2
  norm : Subsystem
  Force_nozzle : Outport
  wires:
  norm/1(|v|) -> Abs1/1
  Abs1/1 -> Switch2/2
  Constant/1 -> Switch1/3
  Switch1/1 -> Activation/1(hit)
  Abs/1 -> Switch3/1, Switch3/2
  Constant1/1 -> Switch/3
  Subsystem/1(value) -> Switch/2
  thrust_vector/1 -> Switch/1
  Activation/1(man_end) -> Subsystem/2(overwrite trigger), Switch2/1
  Switch/1 -> Force_nozzle/1, norm/1(v)
  hit/1 -> Switch1/1, Subsystem/1(input), Scope/1
  ontime/1 -> Abs/1
  Constant2/1 -> Switch3/3
  Switch3/1 -> Activation/2(T_maneuver), Switch1/2

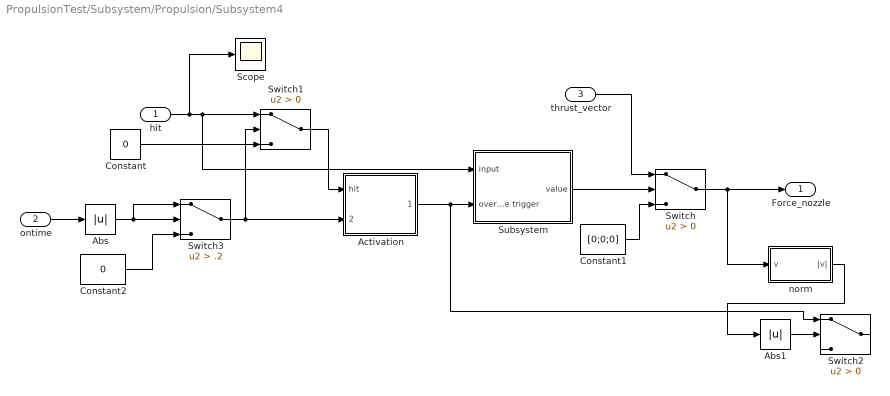
== system PropulsionTest/Subsystem/Propulsion/Subsystem4 ==
  hit : Inport
  ontime : Inport  Port=2
  thrust_vector : Inport  Port=3
  Abs : Abs
  Abs1 : Abs
  Activation : Subsystem
  Constant : Constant  Value=0
  Constant1 : Constant  Value=[0;0;0]
  Constant2 : Constant  Value=0
  Scope : Scope
  Subsystem : Subsystem
  Switch : Switch  Criteria=u2 > Threshold
  Switch1 : Switch  Criteria=u2 > Threshold
  Switch2 : Switch  Criteria=u2 > Threshold
  Switch3 : Switch  Criteria=u2 > Threshold  Threshold=.2
  norm : Subsystem
  Force_nozzle : Outport
  wires:
  Switch3/1 -> Switch1/2, Activation/2(T_maneuver)
  Constant2/1 -> Switch3/3
  ontime/1 -> Abs/1
  hit/1 -> Scope/1, Subsystem/1(input), Switch1/1
  Switch/1 -> norm/1(v), Force_nozzle/1
  Activation/1(man_end) -> Switch2/1, Subsystem/2(overwrite trigger)
  thrust_vector/1 -> Switch/1
  Subsystem/1(value) -> Switch/2
  Constant1/1 -> Switch/3
  Abs/1 -> Switch3/2, Switch3/1
  Switch1/1 -> Activation/1(hit)
  Constant/1 -> Switch1/3
  Abs1/1 -> Switch2/2
  norm/1(|v|) -> Abs1/1

== system PropulsionTest/Subsystem/quat to DCM/Subsystem ==
  In1 : Inport
  3x3 : Reshape  OutputDimensionality=Customize  OutputDimensions=[3,3]
  Demux : Demux  Outputs=3
  Gain : Gain  Gain=-1  SaturateOnIntegerOverflow=on  OutDataTypeStr=Inherit: Same as input  ParamDataTypeStr=Inherit: Same as input
  Gain1 : Gain  Gain=-1  SaturateOnIntegerOverflow=on  OutDataTypeStr=Inherit: Same as input  ParamDataTypeStr=Inherit: Same as input
  Gain2 : Gain  Gain=-1  SaturateOnIntegerOverflow=on  OutDataTypeStr=Inherit: Same as input  ParamDataTypeStr=Inherit: Same as input
  Mux : Mux  Inputs=9
  "diag 0 " : Constant  Value=0
  Out1 : Outport
  wires:
  In1/1 -> Demux/1
  3x3/1 -> Out1/1
  "diag 0 "/1 -> Mux/1, Mux/5, Mux/9
  Mux/1 -> 3x3/1
  Demux/3 -> Mux/2, Gain1/1
  Gain/1 -> Mux/3
  Demux/2 -> Gain/1, Mux/7
  Gain1/1 -> Mux/4
  Demux/1 -> Mux/6, Gain2/1
  Gain2/1 -> Mux/8

== system PropulsionTest/GNC/Follower Maneuver/Optimal Latitude Calc/Enabled Subsystem ==
  r : Inport
  v : Inport  Port=2
  x_tgt : Inport  Port=3
  x_f : Inport  Port=4
  K : Inport  Port=5
  L : Inport  Port=6
  "muE " : Inport  Port=7
  Enable : EnablePort
  MATLAB Function : MATLAB Function  TreatAsAtomicUnit=on
  dV_opt : Outport
  long_opt : Outport  Port=2
  pos_opt : Outport  Port=3
  wires:
  r/1 -> MATLAB Function/1(r)
  v/1 -> MATLAB Function/2(v)
  "muE "/1 -> MATLAB Function/7(muE)
  x_tgt/1 -> MATLAB Function/3(x_t)
  x_f/1 -> MATLAB Function/4(x)
  K/1 -> MATLAB Function/5(K)
  L/1 -> MATLAB Function/6(L)
  MATLAB Function/3(long_opt) -> long_opt/1
  MATLAB Function/1(dV_opt) -> dV_opt/1
  MATLAB Function/2(pos_opt) -> pos_opt/1

== system PropulsionTest/Subsystem/Propulsion/Subsystem1/Activation ==
  note: t_trig + onTime
  note: time of trigger
  note: current time
  hit : Inport
  T_maneuver : Inport  Port=2
  Add : Sum
  Clock : Clock
  Hit Crossing : HitCross
  Subsystem : Subsystem
  Subsystem1 : Subsystem
  Subtract : Sum  Inputs=+-
  man_end : Outport
  wires:
  Subtract/1 -> Hit Crossing/1
  Add/1 -> Subtract/2
  Subsystem/1(value) -> Add/1
  T_maneuver/1 -> Subsystem1/1(input)
  Hit Crossing/1 -> man_end/1
  hit/1 -> Subsystem1/2(overwrite trigger), Subsystem/2(overwrite trigger)
  Clock/1 -> Subtract/1, Subsystem/1(input)
  Subsystem1/1(value) -> Add/2

== system PropulsionTest/Subsystem/Propulsion/Subsystem1/Subsystem ==
  input : Inport
  overwrite trigger : Inport  Port=2
  Data Store Memory : DataStoreMemory  DataStoreName=Mem  ShowAdditionalParam=off
  Data Store Read : DataStoreRead  DataStoreName=Mem  SampleTime=[0,0]  DataStoreElements=Mem
  Data Store Write : DataStoreWrite  DataStoreName=Mem  SampleTime=[0,0]  DataStoreElements=Mem
  Switch : Switch  Criteria=u2 > Threshold
  value : Outport
  wires:
  overwrite trigger/1 -> Switch/2
  Data Store Read/1 -> Switch/3
  Switch/1 -> value/1, Data Store Write/1
  input/1 -> Switch/1

== system PropulsionTest/Subsystem/Propulsion/Subsystem1/norm ==
  v : Inport
  Dot Product : DotProduct  InputSameDT=on  OutDataTypeStr=Inherit: Inherit via internal rule
  Math Function : Math  Operator=sqrt  SaturateOnIntegerOverflow=on
  |v| : Outport
  wires:
  Math Function/1 -> |v|/1
  Dot Product/1 -> Math Function/1
  v/1 -> Dot Product/2, Dot Product/1

== system PropulsionTest/Subsystem/Propulsion/Subsystem2/Activation ==
  note: current time
  note: time of trigger
  note: t_trig + onTime
  hit : Inport
  T_maneuver : Inport  Port=2
  Add : Sum
  Clock : Clock
  Hit Crossing : HitCross
  Subsystem : Subsystem
  Subsystem1 : Subsystem
  Subtract : Sum  Inputs=+-
  man_end : Outport
  wires:
  Subsystem1/1(value) -> Add/2
  Clock/1 -> Subsystem/1(input), Subtract/1
  hit/1 -> Subsystem/2(overwrite trigger), Subsystem1/2(overwrite trigger)
  Hit Crossing/1 -> man_end/1
  T_maneuver/1 -> Subsystem1/1(input)
  Subsystem/1(value) -> Add/1
  Add/1 -> Subtract/2
  Subtract/1 -> Hit Crossing/1

== system PropulsionTest/Subsystem/Propulsion/Subsystem2/Subsystem ==
  input : Inport
  overwrite trigger : Inport  Port=2
  Data Store Memory : DataStoreMemory  DataStoreName=Mem  ShowAdditionalParam=off
  Data Store Read : DataStoreRead  DataStoreName=Mem  SampleTime=[0,0]  DataStoreElements=Mem
  Data Store Write : DataStoreWrite  DataStoreName=Mem  SampleTime=[0,0]  DataStoreElements=Mem
  Switch : Switch  Criteria=u2 > Threshold
  value : Outport
  wires:
  input/1 -> Switch/1
  Switch/1 -> Data Store Write/1, value/1
  Data Store Read/1 -> Switch/3
  overwrite trigger/1 -> Switch/2

== system PropulsionTest/Subsystem/Propulsion/Subsystem2/norm ==
  v : Inport
  Dot Product : DotProduct  InputSameDT=on  OutDataTypeStr=Inherit: Inherit via internal rule
  Math Function : Math  Operator=sqrt  SaturateOnIntegerOverflow=on
  |v| : Outport
  wires:
  v/1 -> Dot Product/1, Dot Product/2
  Dot Product/1 -> Math Function/1
  Math Function/1 -> |v|/1

== system PropulsionTest/Subsystem/Propulsion/Subsystem3/Activation ==
  note: current time
  note: time of trigger
  note: t_trig + onTime
  hit : Inport
  T_maneuver : Inport  Port=2
  Add : Sum
  Clock : Clock
  Hit Crossing : HitCross
  Subsystem : Subsystem
  Subsystem1 : Subsystem
  Subtract : Sum  Inputs=+-
  man_end : Outport
  wires:
  Subsystem1/1(value) -> Add/2
  Clock/1 -> Subsystem/1(input), Subtract/1
  hit/1 -> Subsystem/2(overwrite trigger), Subsystem1/2(overwrite trigger)
  Hit Crossing/1 -> man_end/1
  T_maneuver/1 -> Subsystem1/1(input)
  Subsystem/1(value) -> Add/1
  Add/1 -> Subtract/2
  Subtract/1 -> Hit Crossing/1

== system PropulsionTest/Subsystem/Propulsion/Subsystem3/Subsystem ==
  input : Inport
  overwrite trigger : Inport  Port=2
  Data Store Memory : DataStoreMemory  DataStoreName=Mem  ShowAdditionalParam=off
  Data Store Read : DataStoreRead  DataStoreName=Mem  SampleTime=[0,0]  DataStoreElements=Mem
  Data Store Write : DataStoreWrite  DataStoreName=Mem  SampleTime=[0,0]  DataStoreElements=Mem
  Switch : Switch  Criteria=u2 > Threshold
  value : Outport
  wires:
  input/1 -> Switch/1
  Switch/1 -> Data Store Write/1, value/1
  Data Store Read/1 -> Switch/3
  overwrite trigger/1 -> Switch/2

== system PropulsionTest/Subsystem/Propulsion/Subsystem3/norm ==
  v : Inport
  Dot Product : DotProduct  InputSameDT=on  OutDataTypeStr=Inherit: Inherit via internal rule
  Math Function : Math  Operator=sqrt  SaturateOnIntegerOverflow=on
  |v| : Outport
  wires:
  v/1 -> Dot Product/1, Dot Product/2
  Dot Product/1 -> Math Function/1
  Math Function/1 -> |v|/1

== system PropulsionTest/Subsystem/Propulsion/Subsystem4/Activation ==
  note: t_trig + onTime
  note: time of trigger
  note: current time
  hit : Inport
  T_maneuver : Inport  Port=2
  Add : Sum
  Clock : Clock
  Hit Crossing : HitCross
  Subsystem : Subsystem
  Subsystem1 : Subsystem
  Subtract : Sum  Inputs=+-
  man_end : Outport
  wires:
  Subtract/1 -> Hit Crossing/1
  Add/1 -> Subtract/2
  Subsystem/1(value) -> Add/1
  T_maneuver/1 -> Subsystem1/1(input)
  Hit Crossing/1 -> man_end/1
  hit/1 -> Subsystem1/2(overwrite trigger), Subsystem/2(overwrite trigger)
  Clock/1 -> Subtract/1, Subsystem/1(input)
  Subsystem1/1(value) -> Add/2

== system PropulsionTest/Subsystem/Propulsion/Subsystem4/Subsystem ==
  input : Inport
  overwrite trigger : Inport  Port=2
  Data Store Memory : DataStoreMemory  DataStoreName=Mem  ShowAdditionalParam=off
  Data Store Read : DataStoreRead  DataStoreName=Mem  SampleTime=[0,0]  DataStoreElements=Mem
  Data Store Write : DataStoreWrite  DataStoreName=Mem  SampleTime=[0,0]  DataStoreElements=Mem
  Switch : Switch  Criteria=u2 > Threshold
  value : Outport
  wires:
  overwrite trigger/1 -> Switch/2
  Data Store Read/1 -> Switch/3
  Switch/1 -> value/1, Data Store Write/1
  input/1 -> Switch/1

== system PropulsionTest/Subsystem/Propulsion/Subsystem4/norm ==
  v : Inport
  Dot Product : DotProduct  InputSameDT=on  OutDataTypeStr=Inherit: Inherit via internal rule
  Math Function : Math  Operator=sqrt  SaturateOnIntegerOverflow=on
  |v| : Outport
  wires:
  Math Function/1 -> |v|/1
  Dot Product/1 -> Math Function/1
  v/1 -> Dot Product/2, Dot Product/1

== system PropulsionTest/Subsystem/Propulsion/Subsystem1/Activation/Subsystem ==
  input : Inport
  overwrite trigger : Inport  Port=2
  Data Store Memory : DataStoreMemory  DataStoreName=Mem  ShowAdditionalParam=off
  Data Store Read : DataStoreRead  DataStoreName=Mem  SampleTime=[0,0]  DataStoreElements=Mem
  Data Store Write : DataStoreWrite  DataStoreName=Mem  SampleTime=[0,0]  DataStoreElements=Mem
  Switch : Switch  Criteria=u2 > Threshold
  value : Outport
  wires:
  overwrite trigger/1 -> Switch/2
  Data Store Read/1 -> Switch/3
  Switch/1 -> Data Store Write/1, value/1
  input/1 -> Switch/1

== system PropulsionTest/Subsystem/Propulsion/Subsystem1/Activation/Subsystem1 ==
  input : Inport
  overwrite trigger : Inport  Port=2
  Data Store Memory : DataStoreMemory  DataStoreName=Mem  ShowAdditionalParam=off
  Data Store Read : DataStoreRead  DataStoreName=Mem  SampleTime=[0,0]  DataStoreElements=Mem
  Data Store Write : DataStoreWrite  DataStoreName=Mem  SampleTime=[0,0]  DataStoreElements=Mem
  Switch : Switch  Criteria=u2 > Threshold
  value : Outport
  wires:
  input/1 -> Switch/1
  Switch/1 -> value/1, Data Store Write/1
  Data Store Read/1 -> Switch/3
  overwrite trigger/1 -> Switch/2

== system PropulsionTest/Subsystem/Propulsion/Subsystem2/Activation/Subsystem ==
  input : Inport
  overwrite trigger : Inport  Port=2
  Data Store Memory : DataStoreMemory  DataStoreName=Mem  ShowAdditionalParam=off
  Data Store Read : DataStoreRead  DataStoreName=Mem  SampleTime=[0,0]  DataStoreElements=Mem
  Data Store Write : DataStoreWrite  DataStoreName=Mem  SampleTime=[0,0]  DataStoreElements=Mem
  Switch : Switch  Criteria=u2 > Threshold
  value : Outport
  wires:
  input/1 -> Switch/1
  Switch/1 -> value/1, Data Store Write/1
  Data Store Read/1 -> Switch/3
  overwrite trigger/1 -> Switch/2

== system PropulsionTest/Subsystem/Propulsion/Subsystem2/Activation/Subsystem1 ==
  input : Inport
  overwrite trigger : Inport  Port=2
  Data Store Memory : DataStoreMemory  DataStoreName=Mem  ShowAdditionalParam=off
  Data Store Read : DataStoreRead  DataStoreName=Mem  SampleTime=[0,0]  DataStoreElements=Mem
  Data Store Write : DataStoreWrite  DataStoreName=Mem  SampleTime=[0,0]  DataStoreElements=Mem
  Switch : Switch  Criteria=u2 > Threshold
  value : Outport
  wires:
  overwrite trigger/1 -> Switch/2
  Data Store Read/1 -> Switch/3
  Switch/1 -> Data Store Write/1, value/1
  input/1 -> Switch/1

== system PropulsionTest/Subsystem/Propulsion/Subsystem3/Activation/Subsystem ==
  input : Inport
  overwrite trigger : Inport  Port=2
  Data Store Memory : DataStoreMemory  DataStoreName=Mem  ShowAdditionalParam=off
  Data Store Read : DataStoreRead  DataStoreName=Mem  SampleTime=[0,0]  DataStoreElements=Mem
  Data Store Write : DataStoreWrite  DataStoreName=Mem  SampleTime=[0,0]  DataStoreElements=Mem
  Switch : Switch  Criteria=u2 > Threshold
  value : Outport
  wires:
  input/1 -> Switch/1
  Switch/1 -> value/1, Data Store Write/1
  Data Store Read/1 -> Switch/3
  overwrite trigger/1 -> Switch/2

== system PropulsionTest/Subsystem/Propulsion/Subsystem3/Activation/Subsystem1 ==
  input : Inport
  overwrite trigger : Inport  Port=2
  Data Store Memory : DataStoreMemory  DataStoreName=Mem  ShowAdditionalParam=off
  Data Store Read : DataStoreRead  DataStoreName=Mem  SampleTime=[0,0]  DataStoreElements=Mem
  Data Store Write : DataStoreWrite  DataStoreName=Mem  SampleTime=[0,0]  DataStoreElements=Mem
  Switch : Switch  Criteria=u2 > Threshold
  value : Outport
  wires:
  overwrite trigger/1 -> Switch/2
  Data Store Read/1 -> Switch/3
  Switch/1 -> Data Store Write/1, value/1
  input/1 -> Switch/1

== system PropulsionTest/Subsystem/Propulsion/Subsystem4/Activation/Subsystem ==
  input : Inport
  overwrite trigger : Inport  Port=2
  Data Store Memory : DataStoreMemory  DataStoreName=Mem  ShowAdditionalParam=off
  Data Store Read : DataStoreRead  DataStoreName=Mem  SampleTime=[0,0]  DataStoreElements=Mem
  Data Store Write : DataStoreWrite  DataStoreName=Mem  SampleTime=[0,0]  DataStoreElements=Mem
  Switch : Switch  Criteria=u2 > Threshold
  value : Outport
  wires:
  overwrite trigger/1 -> Switch/2
  Data Store Read/1 -> Switch/3
  Switch/1 -> Data Store Write/1, value/1
  input/1 -> Switch/1

== system PropulsionTest/Subsystem/Propulsion/Subsystem4/Activation/Subsystem1 ==
  input : Inport
  overwrite trigger : Inport  Port=2
  Data Store Memory : DataStoreMemory  DataStoreName=Mem  ShowAdditionalParam=off
  Data Store Read : DataStoreRead  DataStoreName=Mem  SampleTime=[0,0]  DataStoreElements=Mem
  Data Store Write : DataStoreWrite  DataStoreName=Mem  SampleTime=[0,0]  DataStoreElements=Mem
  Switch : Switch  Criteria=u2 > Threshold
  value : Outport
  wires:
  input/1 -> Switch/1
  Switch/1 -> value/1, Data Store Write/1
  Data Store Read/1 -> Switch/3
  overwrite trigger/1 -> Switch/2

== matlab function PropulsionTest/GNC/Follower Maneuver/Impulse Conversion ==
  data: dV_raw input; m_follower input; Imp_filt output size=3; Imp_max input; Imp_min input
function Imp_filt = fcn(dV_raw,m_follower,Imp_max,Imp_min)
%#codegen

Imp_raw = dV_raw*m_follower;

if (norm(Imp_raw)>Imp_max)
    Imp_red=Imp_raw*(Imp_max/norm(Imp_raw));
elseif (norm(Imp_raw)<Imp_min)
    Imp_red=[0;0;0];
else
    Imp_red=Imp_raw;
end

Imp_filt = Imp_red;

== matlab function PropulsionTest/GNC/Follower Maneuver/Optimal Latitude Calc/Enabled Subsystem/MATLAB Function ==
  data: dV_opt output; pos_opt output; long_opt output; r input; v input; x_t input; x input; K input; L input; muE input
function [dV_opt,pos_opt,long_opt] = fcn(r,v,x_t,x,K,L,muE)
%#codegen

z0=[r;v];

E=norm(v)^2/2-muE/norm(r);
a=-muE/(2*E);
T=2*pi/sqrt(muE)*a^(3/2);

options=odeset('AbsTol',1e-12,'RelTol',1e-12);
tspan=linspace(0,T,10000);
[~,zs] = ode45(@orbit1diff,tspan,z0,options,muE,[0;0;0]);

dV_opt = [0;0;0];
pos_opt = [0;0;0];
max_rat=0;
rat=0;
long_opt=0;
N=length(tspan);
x_f=x;
x_diff=x_t-x_f;
% x_diff_hat=x_diff/norm(x_diff);

for i=1:N
    r_f=zs(i,1:3);
    v_f=zs(i,4:6);
    
%     if (abs(dot(r_f,v_f))<perpTol)
%         rat=-999999;
%     end
    
    A=[crs(r_f);
       v_f];

    B=(crs(v_f)*crs(r_f)-crs(crs(r_f)*v_f'))/muE;    
    M=[A;
       B];

    dV_vec=pinv(M)*x_diff;
    dV_opt_sqd=dV_vec'*L*dV_vec;
    dx_vec=M*dV_vec;
    dx_opt_sqd=dx_vec'*K*dx_vec;
    
    rat=dx_opt_sqd/dV_opt_sqd;
    
    if (rat>max_rat)
        max_rat = rat;
        long_opt = atan2(r_f(2),r_f(1));
        pos_opt = r_f';
        dV_opt = dV_vec;
        if (long_opt<0)
            long_opt=long_opt+2*pi;
        end
    end
end
end

== matlab function PropulsionTest/GNC/Target Orbit ==
  data: r_t input; x_tgt output; v_t input; r_f input; v_f input; els_t input; els_f input; muE input; K_F input; match_tol input
function x_tgt = x_target(r_t,v_t,r_f,v_f,els_t,els_f,muE,K_F,match_tol)

h_f = cross(r_f,v_f);
E_f = -muE/(2*els_f(1));
ev_f = cross(v_f,h_f)/muE - r_f/norm(r_f);
x_f_current = [h_f;E_f;ev_f];

h_t = cross(r_t,v_t);
E_t = -muE/(2*els_t(1));
ev_t = cross(v_t,h_t)/muE - r_t/norm(r_t);
x_t_current = [h_t;E_t;ev_t];

if(~orb_matched(x_f_current,x_t_current,K_F,match_tol))
    x_tgt = x_t_current;
else
    pos_diff = r_t-r_f;
    vhat = v_f/norm(v_f);
    dr_vbar = dot(vhat,pos_diff)*vhat;
    along_track_sep = norm(dr_vbar);
    follower_ahead = (dot(vhat,pos_diff) < 0);

    if (norm(r_t-r_f) > 500000)
        if (follower_ahead)
            da_tgt = 500;
        else
            da_tgt = -500;
        end
    else
        [da_tgt,~] = decel_step(along_track_sep,follower_ahead);
    end

    a_tgt = els_t(1) + da_tgt;

    [~,~,x_tgt]=phasing_orbit(els_t,a_tgt,muE);
end

== matlab function PropulsionTest/Position and Velocity to Desired Attitude in Quat/MATLAB Function ==
  data: DCM_be input; q output
function q = fcn(DCM_be)
tr= DCM_be(1,1) + DCM_be(2,2) + DCM_be(3,3);
th= acos((tr-1)/2);
axis= 0.5/sin(th)*[DCM_be(2,3)-DCM_be(3,2);DCM_be(3,1)-DCM_be(1,3);DCM_be(1,2)-DCM_be(2,1)];
q= [axis*sin(th/2);cos(th/2)];
